simulink model "Control_Test"  (R2020a)
settings: Solver=ode1  StartTime=0.0  StopTime=inf  FixedStep=0.001  RelTol=1e-3
InitFcn:
  | COM_config;
  | IO_config;
values from neighbouring files (symbols this model uses):
  AirDensity_kgpm3 = 1.225    [vehicle_controller.mat]
  BatteryCapacity_Wh = 83    [vehicle_controller.mat]
  BatteryInitialEnergy = 58.1    [vehicle_controller.mat]
  BatteryMaxVoltage_V = 96    [vehicle_controller.mat]
  BatteryVoltageCoefficient_x = [0 0.1 0.2 0.3 0.4 0.5 0.6 0.7 0.8 0.9 1]    [vehicle_controller.mat]
  BatteryVoltageCoefficient_y = [0.833333333333 0.85 0.866666666667 0.883333333333 0.9 0.916666666667 0.933333333333 0.95 0.966666666667 0.983333333333 1]    [vehicle_controller.mat]
  BodyInitialSpeed_mps = 0    [vehicle_controller.mat]
  BodyMass_kg = 900    [vehicle_controller.mat]
  CombustionEngineMaxTorque_Nm = 100    [vehicle_controller.mat]
  DragArea_m2 = 4.5    [vehicle_controller.mat]
  DragCoeficient_1 = 0.4    [vehicle_controller.mat]
  FrictionCoefficient_Nsprad = 0.01    [vehicle_controller.mat]
  GearboxRatio_0_1 = 3    [vehicle_controller.mat]
  Ke = 0.1178    [vehicle_controller.mat]
  Kt = 0.668    [vehicle_controller.mat]
  L = looptransfer.Lo    [H_infinity_control_design.m]    (also in LoopShaping.m = G*K; Vehicle_Car_Controller.m = P * C)
  R = 0.141176    [vehicle_controller.mat]
  WheelDiameter_m = 0.5    [vehicle_controller.mat]
undefined symbols (not defined in the file or in its folder): AI_01_range, AI_02_range, AI_03_range, AI_04_range, AI_05_range, AI_06_range, AO_01_max, AO_02_max, AO_03_max, AO_04_max, AO_05_max, AO_06_max, Battery_Voltage_Req, DI_01_mode, DI_01_pullUpDown, DI_02_mode, DI_02_pullUpDown, DI_03_mode, DI_03_pullUpDown, DI_04_mode, DI_04_pullUpDown, DI_05_mode, DI_05_pullUpDown, DI_06_mode, DI_06_pullUpDown, DI_vref_threshold, DO_01_mode, DO_01_outStage, DO_02_mode, DO_02_outStage, DO_03_mode, DO_03_outStage, DO_04_mode, DO_04_outStage, DO_05_mode, DO_05_outStage, DO_06_mode, DO_06_outStage, DO_vref_high, package_period, Serial_Port, Standard_Devices
libraries: simulink x8, sldrtlib x2, simulink_extras x1
(part 2 of 2)

== system Control_Test/Config/Set2/0x1012 ==
  note: 6 Message IDs sent from device to calculator
      | ID 0 means: nothing else to send
  RollingCounter : Inport
  Data Type Conversion{,1..6} (7 alike) : DataTypeConversion
  Data1 : Constant  Value=0x2011
  Data2 : Constant  Value=0x2021
  Data3 : Constant  Value=0x2041
  Data4 : Constant  Value=0x2012
  Data5 : Constant  Value=0x2019
  Data6 : Constant  Value=0x2019
  ID : Constant  Value=0x1012
  Mux : Mux  Inputs=8
  PacketOut : Outport
  wires:
  Mux/1 -> PacketOut/1
  ID/1 -> Data Type Conversion6/1
  Data1/1 -> Data Type Conversion/1
  Data2/1 -> Data Type Conversion1/1
  Data3/1 -> Data Type Conversion2/1
  Data4/1 -> Data Type Conversion3/1
  Data5/1 -> Data Type Conversion4/1
  Data6/1 -> Data Type Conversion5/1
  RollingCounter/1 -> Mux/8
  Data Type Conversion/1 -> Mux/2
  Data Type Conversion1/1 -> Mux/3
  Data Type Conversion2/1 -> Mux/4
  Data Type Conversion3/1 -> Mux/5
  Data Type Conversion4/1 -> Mux/6
  Data Type Conversion5/1 -> Mux/7
  Data Type Conversion6/1 -> Mux/1

== system Control_Test/Config/Set2/0x1013 ==
  note: 6 Message IDs sent from device to calculator
      | ID 0 means: nothing else to send
  RollingCounter : Inport
  Data Type Conversion{,1..6} (7 alike) : DataTypeConversion
  Data1 : Constant  Value=0x2019
  Data2 : Constant  Value=0x2019
  Data{3..6} (4 alike) : Constant  Value=0
  ID : Constant  Value=0x1013
  Mux : Mux  Inputs=8
  PacketOut : Outport
  wires:
  RollingCounter/1 -> Mux/8
  Data6/1 -> Data Type Conversion5/1
  Data5/1 -> Data Type Conversion4/1
  Data4/1 -> Data Type Conversion3/1
  Data3/1 -> Data Type Conversion2/1
  Data2/1 -> Data Type Conversion1/1
  Data1/1 -> Data Type Conversion/1
  ID/1 -> Data Type Conversion6/1
  Mux/1 -> PacketOut/1
  Data Type Conversion5/1 -> Mux/7
  Data Type Conversion4/1 -> Mux/6
  Data Type Conversion3/1 -> Mux/5
  Data Type Conversion2/1 -> Mux/4
  Data Type Conversion1/1 -> Mux/3
  Data Type Conversion/1 -> Mux/2
  Data Type Conversion6/1 -> Mux/1

== system Control_Test/Config/Set2/0x1029 ==
  RollingCounter : Inport
  Data Type Conversion{,1..6} (7 alike) : DataTypeConversion
  Data1 : Constant  Value=AI_01_range
  Data2 : Constant  Value=AI_02_range
  Data3 : Constant  Value=AI_03_range
  Data4 : Constant  Value=AI_04_range
  Data5 : Constant  Value=AI_05_range
  Data6 : Constant  Value=AI_06_range
  ID : Constant  Value=0x1029
  Mux : Mux  Inputs=8
  PacketOut : Outport
  wires:
  Mux/1 -> PacketOut/1
  ID/1 -> Data Type Conversion6/1
  Data1/1 -> Data Type Conversion/1
  Data2/1 -> Data Type Conversion1/1
  Data3/1 -> Data Type Conversion2/1
  Data4/1 -> Data Type Conversion3/1
  Data5/1 -> Data Type Conversion4/1
  Data6/1 -> Data Type Conversion5/1
  RollingCounter/1 -> Mux/8
  Data Type Conversion5/1 -> Mux/7
  Data Type Conversion4/1 -> Mux/6
  Data Type Conversion3/1 -> Mux/5
  Data Type Conversion2/1 -> Mux/4
  Data Type Conversion1/1 -> Mux/3
  Data Type Conversion/1 -> Mux/2
  Data Type Conversion6/1 -> Mux/1

== system Control_Test/Config/Set2/0x1039 ==
  RollingCounter : Inport
  Data Type Conversion{,1..6} (7 alike) : DataTypeConversion
  Data1 : Constant  Value=AO_01_max
  Data2 : Constant  Value=AO_02_max
  Data3 : Constant  Value=AO_03_max
  Data4 : Constant  Value=AO_04_max
  Data5 : Constant  Value=AO_05_max
  Data6 : Constant  Value=AO_06_max
  ID : Constant  Value=0x1039
  Mux : Mux  Inputs=8
  PacketOut : Outport
  wires:
  RollingCounter/1 -> Mux/8
  Data6/1 -> Data Type Conversion5/1
  Data5/1 -> Data Type Conversion4/1
  Data4/1 -> Data Type Conversion3/1
  Data3/1 -> Data Type Conversion2/1
  Data2/1 -> Data Type Conversion1/1
  Data1/1 -> Data Type Conversion/1
  ID/1 -> Data Type Conversion6/1
  Mux/1 -> PacketOut/1
  Data Type Conversion5/1 -> Mux/7
  Data Type Conversion4/1 -> Mux/6
  Data Type Conversion3/1 -> Mux/5
  Data Type Conversion2/1 -> Mux/4
  Data Type Conversion1/1 -> Mux/3
  Data Type Conversion/1 -> Mux/2
  Data Type Conversion6/1 -> Mux/1

== system Control_Test/Config/Set2/0x1047 ==
  RollingCounter : Inport
  Data Type Conversion{,1..6} (7 alike) : DataTypeConversion
  Data1 : Constant  Value=DI_vref_threshold
  Data{2..6} (5 alike) : Constant  Value=0
  ID : Constant  Value=0x1047
  Mux : Mux  Inputs=8
  PacketOut : Outport
  wires:
  Mux/1 -> PacketOut/1
  ID/1 -> Data Type Conversion6/1
  Data1/1 -> Data Type Conversion/1
  Data2/1 -> Data Type Conversion1/1
  Data3/1 -> Data Type Conversion2/1
  Data4/1 -> Data Type Conversion3/1
  Data5/1 -> Data Type Conversion4/1
  Data6/1 -> Data Type Conversion5/1
  RollingCounter/1 -> Mux/8
  Data Type Conversion5/1 -> Mux/7
  Data Type Conversion4/1 -> Mux/6
  Data Type Conversion3/1 -> Mux/5
  Data Type Conversion2/1 -> Mux/4
  Data Type Conversion1/1 -> Mux/3
  Data Type Conversion/1 -> Mux/2
  Data Type Conversion6/1 -> Mux/1

== system Control_Test/Config/Set2/0x1048 ==
  RollingCounter : Inport
  Data Type Conversion{,1..6} (7 alike) : DataTypeConversion
  Data1 : Constant  Value=DI_01_pullUpDown
  Data2 : Constant  Value=DI_02_pullUpDown
  Data3 : Constant  Value=DI_03_pullUpDown
  Data4 : Constant  Value=DI_04_pullUpDown
  Data5 : Constant  Value=DI_05_pullUpDown
  Data6 : Constant  Value=DI_06_pullUpDown
  ID : Constant  Value=0x1048
  Mux : Mux  Inputs=8
  PacketOut : Outport
  wires:
  RollingCounter/1 -> Mux/8
  Data6/1 -> Data Type Conversion5/1
  Data5/1 -> Data Type Conversion4/1
  Data4/1 -> Data Type Conversion3/1
  Data3/1 -> Data Type Conversion2/1
  Data2/1 -> Data Type Conversion1/1
  Data1/1 -> Data Type Conversion/1
  ID/1 -> Data Type Conversion6/1
  Mux/1 -> PacketOut/1
  Data Type Conversion5/1 -> Mux/7
  Data Type Conversion4/1 -> Mux/6
  Data Type Conversion/1 -> Mux/2
  Data Type Conversion1/1 -> Mux/3
  Data Type Conversion2/1 -> Mux/4
  Data Type Conversion3/1 -> Mux/5
  Data Type Conversion6/1 -> Mux/1

== system Control_Test/Config/Set2/0x1049 ==
  RollingCounter : Inport
  Data Type Conversion{,1..6} (7 alike) : DataTypeConversion
  Data1 : Constant  Value=DI_01_mode
  Data2 : Constant  Value=DI_02_mode
  Data3 : Constant  Value=DI_03_mode
  Data4 : Constant  Value=DI_04_mode
  Data5 : Constant  Value=DI_05_mode
  Data6 : Constant  Value=DI_06_mode
  ID : Constant  Value=0x1049
  Mux : Mux  Inputs=8
  PacketOut : Outport
  wires:
  Mux/1 -> PacketOut/1
  ID/1 -> Data Type Conversion6/1
  Data1/1 -> Data Type Conversion/1
  Data2/1 -> Data Type Conversion1/1
  Data3/1 -> Data Type Conversion2/1
  Data4/1 -> Data Type Conversion3/1
  Data5/1 -> Data Type Conversion4/1
  Data6/1 -> Data Type Conversion5/1
  RollingCounter/1 -> Mux/8
  Data Type Conversion/1 -> Mux/2
  Data Type Conversion1/1 -> Mux/3
  Data Type Conversion2/1 -> Mux/4
  Data Type Conversion3/1 -> Mux/5
  Data Type Conversion4/1 -> Mux/6
  Data Type Conversion5/1 -> Mux/7
  Data Type Conversion6/1 -> Mux/1

== system Control_Test/Config/Set2/0x1058 ==
  RollingCounter : Inport
  Data Type Conversion{,1..6} (7 alike) : DataTypeConversion
  Data1 : Constant  Value=DO_vref_high
  Data{2..6} (5 alike) : Constant  Value=0
  ID : Constant  Value=0x1058
  Mux : Mux  Inputs=8
  PacketOut : Outport
  wires:
  RollingCounter/1 -> Mux/8
  Data6/1 -> Data Type Conversion5/1
  Data5/1 -> Data Type Conversion4/1
  Data4/1 -> Data Type Conversion3/1
  Data3/1 -> Data Type Conversion2/1
  Data2/1 -> Data Type Conversion1/1
  Data1/1 -> Data Type Conversion/1
  ID/1 -> Data Type Conversion6/1
  Mux/1 -> PacketOut/1
  Data Type Conversion/1 -> Mux/2
  Data Type Conversion1/1 -> Mux/3
  Data Type Conversion2/1 -> Mux/4
  Data Type Conversion3/1 -> Mux/5
  Data Type Conversion4/1 -> Mux/6
  Data Type Conversion5/1 -> Mux/7
  Data Type Conversion6/1 -> Mux/1

== system Control_Test/Config/Set3/0x1057 ==
  RollingCounter : Inport
  Data Type Conversion{1..7} (7 alike) : DataTypeConversion
  Data1 : Constant  Value=DO_01_outStage
  Data2 : Constant  Value=DO_02_outStage
  Data3 : Constant  Value=DO_03_outStage
  Data4 : Constant  Value=DO_04_outStage
  Data5 : Constant  Value=DO_05_outStage
  Data6 : Constant  Value=DO_06_outStage
  ID : Constant  Value=0x1057
  Mux : Mux  Inputs=8
  PacketOut : Outport
  wires:
  RollingCounter/1 -> Mux/8
  Data6/1 -> Data Type Conversion6/1
  Data5/1 -> Data Type Conversion5/1
  Data4/1 -> Data Type Conversion4/1
  Data3/1 -> Data Type Conversion3/1
  Data2/1 -> Data Type Conversion2/1
  Data1/1 -> Data Type Conversion1/1
  ID/1 -> Data Type Conversion7/1
  Mux/1 -> PacketOut/1
  Data Type Conversion4/1 -> Mux/5
  Data Type Conversion6/1 -> Mux/7
  Data Type Conversion2/1 -> Mux/3
  Data Type Conversion1/1 -> Mux/2
  Data Type Conversion3/1 -> Mux/4
  Data Type Conversion5/1 -> Mux/6
  Data Type Conversion7/1 -> Mux/1

== system Control_Test/Config/Set3/0x1059 ==
  RollingCounter : Inport
  Data Type Conversion{,1..6} (7 alike) : DataTypeConversion
  Data1 : Constant  Value=DO_01_mode
  Data2 : Constant  Value=DO_02_mode
  Data3 : Constant  Value=DO_03_mode
  Data4 : Constant  Value=DO_04_mode
  Data5 : Constant  Value=DO_05_mode
  Data6 : Constant  Value=DO_06_mode
  ID : Constant  Value=0x1059
  Mux : Mux  Inputs=8
  PacketOut : Outport
  wires:
  RollingCounter/1 -> Mux/8
  Data6/1 -> Data Type Conversion5/1
  Data5/1 -> Data Type Conversion4/1
  Data4/1 -> Data Type Conversion3/1
  Data3/1 -> Data Type Conversion2/1
  Data2/1 -> Data Type Conversion1/1
  Data1/1 -> Data Type Conversion/1
  ID/1 -> Data Type Conversion6/1
  Mux/1 -> PacketOut/1
  Data Type Conversion/1 -> Mux/2
  Data Type Conversion1/1 -> Mux/3
  Data Type Conversion2/1 -> Mux/4
  Data Type Conversion3/1 -> Mux/5
  Data Type Conversion4/1 -> Mux/6
  Data Type Conversion5/1 -> Mux/7
  Data Type Conversion6/1 -> Mux/1

== system Control_Test/Config/Set3/Empty2 ==
  RollingCounter : Inport
  Data Type Conversion{1..7} (7 alike) : DataTypeConversion
  Data{1..6} (6 alike) : Constant  Value=0
  ID : Constant  Value=0
  Mux : Mux  Inputs=8
  PacketOut : Outport
  wires:
  Data Type Conversion7/1 -> Mux/1
  Data Type Conversion5/1 -> Mux/6
  Data Type Conversion3/1 -> Mux/4
  Data Type Conversion1/1 -> Mux/2
  Data Type Conversion2/1 -> Mux/3
  Data Type Conversion6/1 -> Mux/7
  Data Type Conversion4/1 -> Mux/5
  Mux/1 -> PacketOut/1
  ID/1 -> Data Type Conversion7/1
  Data1/1 -> Data Type Conversion1/1
  Data2/1 -> Data Type Conversion2/1
  Data3/1 -> Data Type Conversion3/1
  Data4/1 -> Data Type Conversion4/1
  Data5/1 -> Data Type Conversion5/1
  Data6/1 -> Data Type Conversion6/1
  RollingCounter/1 -> Mux/8

== system Control_Test/Config/Set3/Empty3 ==
  RollingCounter : Inport
  Data Type Conversion{1..7} (7 alike) : DataTypeConversion
  Data{1..6} (6 alike) : Constant  Value=0
  ID : Constant  Value=0
  Mux : Mux  Inputs=8
  PacketOut : Outport
  wires:
  RollingCounter/1 -> Mux/8
  Data6/1 -> Data Type Conversion6/1
  Data5/1 -> Data Type Conversion5/1
  Data4/1 -> Data Type Conversion4/1
  Data3/1 -> Data Type Conversion3/1
  Data2/1 -> Data Type Conversion2/1
  Data1/1 -> Data Type Conversion1/1
  ID/1 -> Data Type Conversion7/1
  Mux/1 -> PacketOut/1
  Data Type Conversion4/1 -> Mux/5
  Data Type Conversion6/1 -> Mux/7
  Data Type Conversion2/1 -> Mux/3
  Data Type Conversion1/1 -> Mux/2
  Data Type Conversion3/1 -> Mux/4
  Data Type Conversion5/1 -> Mux/6
  Data Type Conversion7/1 -> Mux/1

== system Control_Test/Config/Set3/Empty4 ==
  RollingCounter : Inport
  Data Type Conversion{1..7} (7 alike) : DataTypeConversion
  Data{1..6} (6 alike) : Constant  Value=0
  ID : Constant  Value=0
  Mux : Mux  Inputs=8
  PacketOut : Outport
  wires:
  Data Type Conversion7/1 -> Mux/1
  Data Type Conversion5/1 -> Mux/6
  Data Type Conversion3/1 -> Mux/4
  Data Type Conversion1/1 -> Mux/2
  Data Type Conversion2/1 -> Mux/3
  Data Type Conversion6/1 -> Mux/7
  Data Type Conversion4/1 -> Mux/5
  Mux/1 -> PacketOut/1
  ID/1 -> Data Type Conversion7/1
  Data1/1 -> Data Type Conversion1/1
  Data2/1 -> Data Type Conversion2/1
  Data3/1 -> Data Type Conversion3/1
  Data4/1 -> Data Type Conversion4/1
  Data5/1 -> Data Type Conversion5/1
  Data6/1 -> Data Type Conversion6/1
  RollingCounter/1 -> Mux/8

== system Control_Test/Config/Set3/Empty5 ==
  RollingCounter : Inport
  Data Type Conversion{1..7} (7 alike) : DataTypeConversion
  Data{1..6} (6 alike) : Constant  Value=0
  ID : Constant  Value=0
  Mux : Mux  Inputs=8
  PacketOut : Outport
  wires:
  RollingCounter/1 -> Mux/8
  Data6/1 -> Data Type Conversion6/1
  Data5/1 -> Data Type Conversion5/1
  Data4/1 -> Data Type Conversion4/1
  Data3/1 -> Data Type Conversion3/1
  Data2/1 -> Data Type Conversion2/1
  Data1/1 -> Data Type Conversion1/1
  ID/1 -> Data Type Conversion7/1
  Mux/1 -> PacketOut/1
  Data Type Conversion4/1 -> Mux/5
  Data Type Conversion6/1 -> Mux/7
  Data Type Conversion2/1 -> Mux/3
  Data Type Conversion1/1 -> Mux/2
  Data Type Conversion3/1 -> Mux/4
  Data Type Conversion5/1 -> Mux/6
  Data Type Conversion7/1 -> Mux/1

== system Control_Test/Config/Set3/Empty6 ==
  RollingCounter : Inport
  Data Type Conversion{1..7} (7 alike) : DataTypeConversion
  Data{1..6} (6 alike) : Constant  Value=0
  ID : Constant  Value=0
  Mux : Mux  Inputs=8
  PacketOut : Outport
  wires:
  Data Type Conversion7/1 -> Mux/1
  Data Type Conversion5/1 -> Mux/6
  Data Type Conversion3/1 -> Mux/4
  Data Type Conversion1/1 -> Mux/2
  Data Type Conversion2/1 -> Mux/3
  Data Type Conversion6/1 -> Mux/7
  Data Type Conversion4/1 -> Mux/5
  Mux/1 -> PacketOut/1
  ID/1 -> Data Type Conversion7/1
  Data1/1 -> Data Type Conversion1/1
  Data2/1 -> Data Type Conversion2/1
  Data3/1 -> Data Type Conversion3/1
  Data4/1 -> Data Type Conversion4/1
  Data5/1 -> Data Type Conversion5/1
  Data6/1 -> Data Type Conversion6/1
  RollingCounter/1 -> Mux/8

== system Control_Test/Config/Set3/Empty7 ==
  RollingCounter : Inport
  Data Type Conversion{1..7} (7 alike) : DataTypeConversion
  Data{1..6} (6 alike) : Constant  Value=0
  ID : Constant  Value=0
  Mux : Mux  Inputs=8
  PacketOut : Outport
  wires:
  RollingCounter/1 -> Mux/8
  Data6/1 -> Data Type Conversion6/1
  Data5/1 -> Data Type Conversion5/1
  Data4/1 -> Data Type Conversion4/1
  Data3/1 -> Data Type Conversion3/1
  Data2/1 -> Data Type Conversion2/1
  Data1/1 -> Data Type Conversion1/1
  ID/1 -> Data Type Conversion7/1
  Mux/1 -> PacketOut/1
  Data Type Conversion4/1 -> Mux/5
  Data Type Conversion6/1 -> Mux/7
  Data Type Conversion2/1 -> Mux/3
  Data Type Conversion1/1 -> Mux/2
  Data Type Conversion3/1 -> Mux/4
  Data Type Conversion5/1 -> Mux/6
  Data Type Conversion7/1 -> Mux/1

== system Control_Test/Running/InSet/AI ==
  PacketIn : Inport
  Bus Creator : BusCreator  Inputs=6
  Demux : Demux  Outputs=8
  RollingCounter : Outport
  ID : Outport  Port=2
  AI : Outport  Port=3
  wires:
  Demux/7 -> Bus Creator/6  "AI_06"
  Demux/6 -> Bus Creator/5  "AI_05"
  Demux/5 -> Bus Creator/4  "AI_04"
  Demux/4 -> Bus Creator/3  "AI_03"
  Demux/3 -> Bus Creator/2  "AI_02"
  Demux/2 -> Bus Creator/1  "AI_01"
  Demux/1 -> ID/1
  Demux/8 -> RollingCounter/1
  PacketIn/1 -> Demux/1
  Bus Creator/1 -> AI/1

== system Control_Test/Running/InSet/BatteryVoltage ==
  PacketIn : Inport
  Demux : Demux  Outputs=8
  Terminator{1..5} (5 alike) : Terminator
  RollingCounter : Outport
  ID : Outport  Port=2
  Battery_Voltage : Outport  Port=3
  wires:
  Demux/7 -> Terminator5/1
  Demux/6 -> Terminator4/1
  Demux/5 -> Terminator3/1
  Demux/4 -> Terminator2/1
  Demux/3 -> Terminator1/1
  Demux/2 -> Battery_Voltage/1
  Demux/1 -> ID/1
  Demux/8 -> RollingCounter/1
  PacketIn/1 -> Demux/1

== system Control_Test/Running/InSet/DI ==
  PacketIn : Inport
  Bus Creator : BusCreator  Inputs=6
  Demux : Demux  Outputs=8
  RollingCounter : Outport
  ID : Outport  Port=2
  DI : Outport  Port=3
  wires:
  Bus Creator/1 -> DI/1
  PacketIn/1 -> Demux/1
  Demux/8 -> RollingCounter/1
  Demux/1 -> ID/1
  Demux/2 -> Bus Creator/1  "DI_01"
  Demux/3 -> Bus Creator/2  "DI_02"
  Demux/4 -> Bus Creator/3  "DI_03"
  Demux/5 -> Bus Creator/4  "DI_04"
  Demux/6 -> Bus Creator/5  "DI_05"
  Demux/7 -> Bus Creator/6  "DI_06"

== system Control_Test/Running/InSet/Empty2 ==
  PacketIn : Inport
  Demux : Demux  Outputs=8
  Terminator{,1..5} (6 alike) : Terminator
  RollingCounter : Outport
  ID : Outport  Port=2
  wires:
  Demux/7 -> Terminator5/1
  Demux/6 -> Terminator4/1
  Demux/5 -> Terminator3/1
  Demux/4 -> Terminator2/1
  Demux/3 -> Terminator1/1
  Demux/2 -> Terminator/1
  Demux/1 -> ID/1
  Demux/8 -> RollingCounter/1
  PacketIn/1 -> Demux/1

== system Control_Test/Running/InSet/Empty3 ==
  PacketIn : Inport
  Demux : Demux  Outputs=8
  Terminator{,1..5} (6 alike) : Terminator
  RollingCounter : Outport
  ID : Outport  Port=2
  wires:
  PacketIn/1 -> Demux/1
  Demux/8 -> RollingCounter/1
  Demux/1 -> ID/1
  Demux/2 -> Terminator/1
  Demux/3 -> Terminator1/1
  Demux/4 -> Terminator2/1
  Demux/5 -> Terminator3/1
  Demux/6 -> Terminator4/1
  Demux/7 -> Terminator5/1

== system Control_Test/Running/InSet/Empty4 ==
  PacketIn : Inport
  Demux : Demux  Outputs=8
  Terminator{,1..5} (6 alike) : Terminator
  RollingCounter : Outport
  ID : Outport  Port=2
  wires:
  PacketIn/1 -> Demux/1
  Demux/8 -> RollingCounter/1
  Demux/1 -> ID/1
  Demux/2 -> Terminator/1
  Demux/3 -> Terminator1/1
  Demux/4 -> Terminator2/1
  Demux/5 -> Terminator3/1
  Demux/6 -> Terminator4/1
  Demux/7 -> Terminator5/1

== system Control_Test/Running/InSet/Empty5 ==
  PacketIn : Inport
  Demux : Demux  Outputs=8
  Terminator{,1..5} (6 alike) : Terminator
  RollingCounter : Outport
  ID : Outport  Port=2
  wires:
  Demux/7 -> Terminator5/1
  Demux/6 -> Terminator4/1
  Demux/5 -> Terminator3/1
  Demux/4 -> Terminator2/1
  Demux/3 -> Terminator1/1
  Demux/2 -> Terminator/1
  Demux/1 -> ID/1
  Demux/8 -> RollingCounter/1
  PacketIn/1 -> Demux/1

== system Control_Test/Running/InSet/Empty6 ==
  PacketIn : Inport
  Demux : Demux  Outputs=8
  Terminator{,1..5} (6 alike) : Terminator
  RollingCounter : Outport
  ID : Outport  Port=2
  wires:
  Demux/7 -> Terminator5/1
  Demux/6 -> Terminator4/1
  Demux/5 -> Terminator3/1
  Demux/4 -> Terminator2/1
  Demux/3 -> Terminator1/1
  Demux/2 -> Terminator/1
  Demux/1 -> ID/1
  Demux/8 -> RollingCounter/1
  PacketIn/1 -> Demux/1

== system Control_Test/Running/Model/AirDrag ==
  VehicleSpeed_mps : Inport
  " " : Constant  Value=0.5
  AirDensity_kgpm3 : Constant  Value=AirDensity_kgpm3
  DragArea_m2 : Constant  Value=DragArea_m2
  DragCoeficient_1 : Constant  Value=DragCoeficient_1
  Product : Product  Inputs=5
  Square : Math  Operator=square  SaturateOnIntegerOverflow=on
  AirDragForce_N : Outport
  wires:
  VehicleSpeed_mps/1 -> Square/1
  Square/1 -> Product/5
  DragArea_m2/1 -> Product/3
  AirDensity_kgpm3/1 -> Product/4
  DragCoeficient_1/1 -> Product/2
  " "/1 -> Product/1
  Product/1 -> AirDragForce_N/1

== system Control_Test/Running/Model/Battery ==
  BatteryCurrent_A : Inport
  1-D Lookup Table : Lookup_n-D  NumberOfTableDimensions=1  BreakpointsForDimension1=BatteryVoltageCoefficient_x  Table=BatteryVoltageCoefficient_y  InternalRulePriority=Speed  RndMeth=Simplest  InputSameDT=on
  BatteryCapacity_Wh : Constant  Value=BatteryCapacity_Wh
  BatteryMaxVoltage_V : Constant  Value=BatteryMaxVoltage_V
  Gain : Gain  Gain=-1
  Gain1 : Gain  Gain=1/3600
  Integrator : Integrator  InitialCondition=BatteryInitialEnergy
  Product : Product
  Product1 : Product  Inputs=*/
  Product2 : Product
  BatteryVoltage_V : Outport
  wires:
  BatteryCurrent_A/1 -> Product2/1  "BatteryCurrent_A"
  Product/1 -> Product2/2, BatteryVoltage_V/1  "BatteryVoltage_V"
  Integrator/1 -> Product1/1  "Energy_Wh"
  1-D Lookup Table/1 -> Product/2  "VoltageCoeficient_0_1"
  BatteryMaxVoltage_V/1 -> Product/1
  BatteryCapacity_Wh/1 -> Product1/2
  Product1/1 -> 1-D Lookup Table/1  "StateOfCharge_0_1"
  Product2/1 -> Gain/1
  Gain/1 -> Gain1/1
  Gain1/1 -> Integrator/1

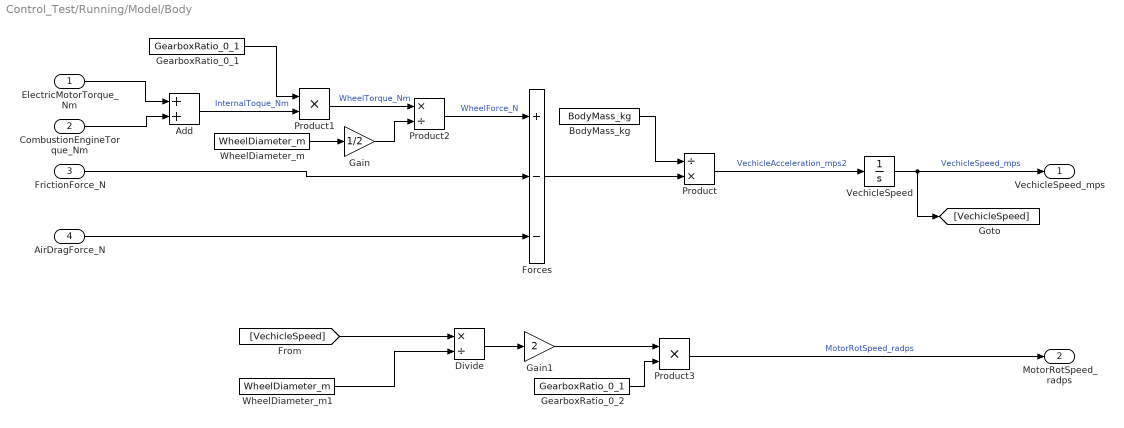
== system Control_Test/Running/Model/Body ==
  ElectricMotorTorque_Nm : Inport
  CombustionEngineTorque_Nm : Inport  Port=2
  FrictionForce_N : Inport  Port=3
  AirDragForce_N : Inport  Port=4
  Add : Sum
  BodyMass_kg : Constant  Value=BodyMass_kg
  Divide : Product  Inputs=*/
  Forces : Sum  Inputs=+--
  Gain : Gain  Gain=1/2
  Gain1 : Gain  Gain=2
  GearboxRatio_0_1 : Constant  Value=GearboxRatio_0_1
  GearboxRatio_0_2 : Constant  Value=GearboxRatio_0_1
  Product : Product  Inputs=/*
  Product1 : Product
  Product2 : Product  Inputs=*/
  Product3 : Product  Inputs=**
  VechicleSpeed : Integrator  InitialCondition=BodyInitialSpeed_mps
  WheelDiameter_m : Constant  Value=WheelDiameter_m
  WheelDiameter_m1 : Constant  Value=WheelDiameter_m
  VechicleSpeed_mps : Outport
  MotorRotSpeed_radps : Outport  Port=2
  wires:
  VechicleSpeed/1 -> [VechicleSpeed], VechicleSpeed_mps/1  "VechicleSpeed_mps"
  Product/1 -> VechicleSpeed/1  "VechicleAcceleration_mps2"
  BodyMass_kg/1 -> Product/1
  Forces/1 -> Product/2
  AirDragForce_N/1 -> Forces/3
  FrictionForce_N/1 -> Forces/2
  ElectricMotorTorque_Nm/1 -> Add/1
  CombustionEngineTorque_Nm/1 -> Add/2
  Add/1 -> Product1/2  "InternalToque_Nm"
  GearboxRatio_0_1/1 -> Product1/1
  Product1/1 -> Product2/1  "WheelTorque_Nm"
  WheelDiameter_m/1 -> Gain/1
  Product2/1 -> Forces/1  "WheelForce_N"
  Gain/1 -> Product2/2
  [VechicleSpeed] -> Divide/1
  WheelDiameter_m1/1 -> Divide/2
  Divide/1 -> Gain1/1
  Gain1/1 -> Product3/1
  GearboxRatio_0_2/1 -> Product3/2
  Product3/1 -> MotorRotSpeed_radps/1  "MotorRotSpeed_radps"

== system Control_Test/Running/Model/CombustionEngine ==
  CombustionEngineStart_1 : Inport
  Gain : Gain  Gain=CombustionEngineMaxTorque_Nm
  Transfer Fcn : TransferFcn  Denominator=[1 1]
  CombustionEngineTorque_Nm : Outport
  wires:
  Transfer Fcn/1 -> CombustionEngineTorque_Nm/1
  CombustionEngineStart_1/1 -> Gain/1
  Gain/1 -> Transfer Fcn/1

== system Control_Test/Running/Model/Driver ==
  BatteryVoltage_V : Inport
  DutyCycle_1 : Inport  Port=2
  Direction_1 : Inport  Port=3
  MotorCurrent_A : Inport  Port=4
  Product : Product
  Product1 : Product
  Product2 : Product
  MotorVoltage_V : Outport
  BatteryCurrent_A : Outport  Port=2
  wires:
  BatteryVoltage_V/1 -> Product/1
  Product/1 -> MotorVoltage_V/1
  Product2/1 -> Product1/1, Product/2
  MotorCurrent_A/1 -> Product1/2
  Product1/1 -> BatteryCurrent_A/1
  DutyCycle_1/1 -> Product2/1
  Direction_1/1 -> Product2/2

== system Control_Test/Running/Model/ElectricMotor ==
  MotorRotSpeed_radps : Inport
  MotorVoltage_V : Inport  Port=2
  Add : Sum  Inputs=-+-
  Constant : Constant  Value=Kt
  Constant1 : Constant  Value=L
  Constant2 : Constant  Value=R
  Constant3 : Constant  Value=Ke
  Integrator : Integrator
  Product : Product
  Product1 : Product  Inputs=*/
  Product2 : Product
  Product3 : Product
  Scope : Scope
  MotorTorque_Nm : Outport
  MotorCurrent_A : Outport  Port=2
  wires:
  Product/1 -> MotorTorque_Nm/1
  Integrator/1 -> MotorCurrent_A/1, Product2/2, Scope/1, Product/2  "MotorCurrent_A"
  Constant/1 -> Product/1
  Product1/1 -> Integrator/1
  Constant1/1 -> Product1/2
  Add/1 -> Product1/1
  Product2/1 -> Add/3
  Constant2/1 -> Product2/1
  MotorVoltage_V/1 -> Add/2
  Constant3/1 -> Product3/1
  Product3/1 -> Add/1
  MotorRotSpeed_radps/1 -> Product3/2

== system Control_Test/Running/Model/Frictions ==
  MotorSpeed_radps : Inport
  FrictionCoefficient_Nsprad : Constant  Value=FrictionCoefficient_Nsprad
  Product : Product
  FrictionForce_N : Outport
  wires:
  Product/1 -> FrictionForce_N/1
  MotorSpeed_radps/1 -> Product/2
  FrictionCoefficient_Nsprad/1 -> Product/1

== system Control_Test/Running/Model/Subsystem ==
  In1 : Inport
  Constant : Constant  Value=00  OutDataTypeStr=Inherit: Inherit via back propagation
  IsNaN : RelationalOperator  Operator=isNaN  OutDataTypeStr=boolean  RndMeth=Simplest
  Switch : Switch  Criteria=u2 > Threshold
  DutyCycle_1 : Outport
  wires:
  Switch/1 -> DutyCycle_1/1
  In1/1 -> IsNaN/1, Switch/3
  IsNaN/1 -> Switch/2
  Constant/1 -> Switch/1

== system Control_Test/Running/Model/Subsystem1 ==
  In1 : Inport
  Constant : Constant  Value=00  OutDataTypeStr=Inherit: Inherit via back propagation
  IsNaN : RelationalOperator  Operator=isNaN  OutDataTypeStr=boolean  RndMeth=Simplest
  Switch : Switch  Criteria=u2 > Threshold
  Direction_1 : Outport
  wires:
  Constant/1 -> Switch/1
  IsNaN/1 -> Switch/2
  In1/1 -> Switch/3, IsNaN/1
  Switch/1 -> Direction_1/1

== system Control_Test/Running/Model/Subsystem2 ==
  In1 : Inport
  Constant : Constant  Value=00  OutDataTypeStr=Inherit: Inherit via back propagation
  IsNaN : RelationalOperator  Operator=isNaN  OutDataTypeStr=boolean  RndMeth=Simplest
  Switch : Switch  Criteria=u2 > Threshold
  Direction_1 : Outport
  wires:
  Switch/1 -> Direction_1/1
  In1/1 -> IsNaN/1, Switch/3
  IsNaN/1 -> Switch/2
  Constant/1 -> Switch/1

== system Control_Test/Running/ModelInputs/Subsystem2 ==
  <AI> : Inport
  Bus Selector1 : BusSelector  OutputSignals=AI_01,AI_02,AI_03,AI_04,AI_05,AI_06
  Data Type Conversion{,1..5} (6 alike) : DataTypeConversion
  tag scope: AI_01=scoped, AI_02=scoped, AI_03=scoped, AI_04=scoped, AI_05=scoped, AI_06=scoped
  wires:
  Bus Selector1/4 -> Data Type Conversion3/1  "<AI_04>"
  Bus Selector1/3 -> Data Type Conversion2/1  "<AI_03>"
  Bus Selector1/6 -> Data Type Conversion5/1  "<AI_06>"
  Bus Selector1/2 -> Data Type Conversion1/1  "<AI_02>"
  Bus Selector1/1 -> Data Type Conversion/1  "<AI_01>"
  <AI>/1 -> Bus Selector1/1
  Data Type Conversion/1 -> [AI_01]
  Bus Selector1/5 -> Data Type Conversion4/1  "<AI_05>"
  Data Type Conversion1/1 -> [AI_02]
  Data Type Conversion2/1 -> [AI_03]
  Data Type Conversion3/1 -> [AI_04]
  Data Type Conversion4/1 -> [AI_05]
  Data Type Conversion5/1 -> [AI_06]

== system Control_Test/Running/ModelInputs/Subsystem3 ==
  <DI> : Inport
  Bus Selector2 : BusSelector  OutputSignals=DI_01,DI_02,DI_03,DI_04,DI_05,DI_06
  Data Type Conversion{,1..5} (6 alike) : DataTypeConversion
  tag scope: DI_01=scoped, DI_02=scoped, DI_03=scoped, DI_04=scoped, DI_05=scoped, DI_06=scoped
  wires:
  Bus Selector2/3 -> Data Type Conversion2/1  "<DI_03>"
  Bus Selector2/6 -> Data Type Conversion5/1  "<DI_06>"
  Bus Selector2/2 -> Data Type Conversion1/1  "<DI_02>"
  Bus Selector2/1 -> Data Type Conversion/1  "<DI_01>"
  Bus Selector2/4 -> Data Type Conversion3/1  "<DI_04>"
  Bus Selector2/5 -> Data Type Conversion4/1  "<DI_05>"
  <DI>/1 -> Bus Selector2/1
  Data Type Conversion/1 -> [DI_01]
  Data Type Conversion3/1 -> [DI_04]
  Data Type Conversion4/1 -> [DI_05]
  Data Type Conversion5/1 -> [DI_06]
  Data Type Conversion1/1 -> [DI_02]
  Data Type Conversion2/1 -> [DI_03]

== system Control_Test/Running/ModelOutputs/AO ==
  Bus Creator : BusCreator  Inputs=6
  Data Type Conversion{,1..5} (6 alike) : DataTypeConversion  OutDataTypeStr=uint32
  AO : Outport
  wires:
  Data Type Conversion1/1 -> Bus Creator/2  "AO_02"
  Data Type Conversion3/1 -> Bus Creator/4  "AO_04"
  Data Type Conversion4/1 -> Bus Creator/5  "AO_05"
  [AO_06] -> Data Type Conversion5/1  "AO_06"
  Data Type Conversion2/1 -> Bus Creator/3  "AO_03"
  Data Type Conversion/1 -> Bus Creator/1  "AO_01"
  Bus Creator/1 -> AO/1  "AO"
  Data Type Conversion5/1 -> Bus Creator/6  "AO_06"
  [AO_05] -> Data Type Conversion4/1  "AO_05"
  [AO_01] -> Data Type Conversion/1  "AO_01"
  [AO_02] -> Data Type Conversion1/1  "AO_02"
  [AO_03] -> Data Type Conversion2/1  "AO_03"
  [AO_04] -> Data Type Conversion3/1  "AO_04"

== system Control_Test/Running/ModelOutputs/DO_Duty ==
  Bus Creator3 : BusCreator  Inputs=6
  Data Type Conversion{,1..5} (6 alike) : DataTypeConversion  OutDataTypeStr=uint32
  DO_Duty : Outport
  wires:
  Data Type Conversion1/1 -> Bus Creator3/2  "DO_02_Duty"
  Data Type Conversion5/1 -> Bus Creator3/6  "DO_06_Duty"
  Data Type Conversion/1 -> Bus Creator3/1  "DO_01_Duty"
  Data Type Conversion4/1 -> Bus Creator3/5  "DO_05_Duty"
  Data Type Conversion2/1 -> Bus Creator3/3  "DO_03_Duty"
  Data Type Conversion3/1 -> Bus Creator3/4  "DO_04_Duty"
  Bus Creator3/1 -> DO_Duty/1  "DO_Duty"
  [DO_01_Duty] -> Data Type Conversion/1  "DO_01_Duty"
  [DO_02_Duty] -> Data Type Conversion1/1  "DO_02_Duty"
  [DO_03_Duty] -> Data Type Conversion2/1  "DO_03_Duty"
  [DO_04_Duty] -> Data Type Conversion3/1  "DO_04_Duty"
  [DO_05_Duty] -> Data Type Conversion4/1  "DO_05_Duty"
  [DO_06_Duty] -> Data Type Conversion5/1  "DO_06_Duty"

== system Control_Test/Running/ModelOutputs/DO_Freq ==
  Bus Creator2 : BusCreator  Inputs=6
  Data Type Conversion{,1..5} (6 alike) : DataTypeConversion  OutDataTypeStr=uint32
  DO_Freq : Outport
  wires:
  Data Type Conversion/1 -> Bus Creator2/1  "DO_01_Freq"
  Data Type Conversion3/1 -> Bus Creator2/4  "DO_04_Freq"
  Bus Creator2/1 -> DO_Freq/1  "DO_Freq"
  Data Type Conversion4/1 -> Bus Creator2/5  "DO_05_Freq"
  Data Type Conversion5/1 -> Bus Creator2/6  "DO_06_Freq"
  Data Type Conversion2/1 -> Bus Creator2/3  "DO_03_Freq"
  Data Type Conversion1/1 -> Bus Creator2/2  "DO_02_Freq"
  [DO_01_Freq] -> Data Type Conversion/1  "DO_01_Freq"
  [DO_02_Freq] -> Data Type Conversion1/1  "DO_02_Freq"
  [DO_03_Freq] -> Data Type Conversion2/1  "DO_03_Freq"
  [DO_04_Freq] -> Data Type Conversion3/1  "DO_04_Freq"
  [DO_05_Freq] -> Data Type Conversion4/1  "DO_05_Freq"
  [DO_06_Freq] -> Data Type Conversion5/1  "DO_06_Freq"

== system Control_Test/Running/ModelOutputs/DO_Level ==
  Bus Creator1 : BusCreator  Inputs=6
  Data Type Conversion{,1..5} (6 alike) : DataTypeConversion  OutDataTypeStr=uint32
  DO_Level : Outport
  wires:
  Data Type Conversion1/1 -> Bus Creator1/2  "DO_02_Level"
  Bus Creator1/1 -> DO_Level/1  "DO_Level"
  Data Type Conversion2/1 -> Bus Creator1/3  "DO_03_Level"
  Data Type Conversion4/1 -> Bus Creator1/5  "DO_05_Level"
  Data Type Conversion3/1 -> Bus Creator1/4  "DO_04_Level"
  Data Type Conversion/1 -> Bus Creator1/1  "DO_01_Level"
  Data Type Conversion5/1 -> Bus Creator1/6  "DO_06_Level"
  [DO_04] -> Data Type Conversion3/1  "DO_04_Level"
  [DO_03] -> Data Type Conversion2/1  "DO_03_Level"
  [DO_02] -> Data Type Conversion1/1  "DO_02_Level"
  [DO_01] -> Data Type Conversion/1  "DO_01_Level"
  [DO_05] -> Data Type Conversion4/1  "DO_05_Level"
  [DO_06] -> Data Type Conversion5/1  "DO_06_Level"

== system Control_Test/Running/OutSet/0x1019 ==
  RollingCounter : Inport
  Battery_Active : Inport  Port=2
  Data Type Conversion{1..7} (7 alike) : DataTypeConversion
  Data2 : Constant  Value=Battery_Voltage_Req
  Data{3..6} (4 alike) : Constant  Value=0
  ID : Constant  Value=0x1019
  Mux : Mux  Inputs=8
  PacketOut : Outport
  wires:
  RollingCounter/1 -> Mux/8
  Data6/1 -> Data Type Conversion6/1
  Data5/1 -> Data Type Conversion5/1
  Data4/1 -> Data Type Conversion4/1
  Data3/1 -> Data Type Conversion3/1
  Data2/1 -> Data Type Conversion2/1
  Battery_Active/1 -> Data Type Conversion1/1
  ID/1 -> Data Type Conversion7/1
  Mux/1 -> PacketOut/1
  Data Type Conversion4/1 -> Mux/5
  Data Type Conversion6/1 -> Mux/7
  Data Type Conversion2/1 -> Mux/3
  Data Type Conversion1/1 -> Mux/2
  Data Type Conversion3/1 -> Mux/4
  Data Type Conversion5/1 -> Mux/6
  Data Type Conversion7/1 -> Mux/1

== system Control_Test/Running/OutSet/0x1031 ==
  RollingCounter : Inport
  DAC : Inport  Port=2
  Bus Selector : BusSelector  OutputSignals=AO_01,AO_02,AO_03,AO_04,AO_05,AO_06
  ID : Constant  Value=0x1031  OutDataTypeStr=uint32
  Mux : Mux  Inputs=8
  PacketOut : Outport
  wires:
  Mux/1 -> PacketOut/1
  ID/1 -> Mux/1
  RollingCounter/1 -> Mux/8
  DAC/1 -> Bus Selector/1
  Bus Selector/1 -> Mux/2  "<AO_01>"
  Bus Selector/2 -> Mux/3  "<AO_02>"
  Bus Selector/3 -> Mux/4  "<AO_03>"
  Bus Selector/4 -> Mux/5  "<AO_04>"
  Bus Selector/5 -> Mux/6  "<AO_05>"
  Bus Selector/6 -> Mux/7  "<AO_06>"

== system Control_Test/Running/OutSet/0x1051 ==
  RollingCounter : Inport
  DO_Level : Inport  Port=2
  Bus Selector : BusSelector  OutputSignals=DO_01_Level,DO_02_Level,DO_03_Level,DO_04_Level,DO_05_Level,DO_06_Level
  ID : Constant  Value=0x1051  OutDataTypeStr=uint32
  Mux : Mux  Inputs=8
  PacketOut : Outport
  wires:
  RollingCounter/1 -> Mux/8
  Bus Selector/5 -> Mux/6  "<DO_05_Level>"
  Bus Selector/3 -> Mux/4  "<DO_03_Level>"
  Bus Selector/1 -> Mux/2  "<DO_01_Level>"
  ID/1 -> Mux/1
  Mux/1 -> PacketOut/1
  DO_Level/1 -> Bus Selector/1
  Bus Selector/2 -> Mux/3  "<DO_02_Level>"
  Bus Selector/4 -> Mux/5  "<DO_04_Level>"
  Bus Selector/6 -> Mux/7  "<DO_06_Level>"

== system Control_Test/Running/OutSet/0x1052 ==
  RollingCounter : Inport
  DO_Freq : Inport  Port=2
  Bus Selector : BusSelector  OutputSignals=DO_01_Freq,DO_02_Freq,DO_03_Freq,DO_04_Freq,DO_05_Freq,DO_06_Freq
  ID : Constant  Value=0x1052  OutDataTypeStr=uint32
  Mux : Mux  Inputs=8
  PacketOut : Outport
  wires:
  Mux/1 -> PacketOut/1
  ID/1 -> Mux/1
  RollingCounter/1 -> Mux/8
  DO_Freq/1 -> Bus Selector/1
  Bus Selector/1 -> Mux/2  "<DO_01_Freq>"
  Bus Selector/2 -> Mux/3  "<DO_02_Freq>"
  Bus Selector/3 -> Mux/4  "<DO_03_Freq>"
  Bus Selector/4 -> Mux/5  "<DO_04_Freq>"
  Bus Selector/5 -> Mux/6  "<DO_05_Freq>"
  Bus Selector/6 -> Mux/7  "<DO_06_Freq>"

== system Control_Test/Running/OutSet/0x1053 ==
  RollingCounter : Inport
  DO_Duty : Inport  Port=2
  Bus Selector : BusSelector  OutputSignals=DO_01_Duty,DO_02_Duty,DO_03_Duty,DO_04_Duty,DO_05_Duty,DO_06_Duty
  ID : Constant  Value=0x1053  OutDataTypeStr=uint32
  Mux : Mux  Inputs=8
  PacketOut : Outport
  wires:
  RollingCounter/1 -> Mux/8
  ID/1 -> Mux/1
  Mux/1 -> PacketOut/1
  DO_Duty/1 -> Bus Selector/1
  Bus Selector/1 -> Mux/2  "<DO_01_Duty>"
  Bus Selector/2 -> Mux/3  "<DO_02_Duty>"
  Bus Selector/3 -> Mux/4  "<DO_03_Duty>"
  Bus Selector/4 -> Mux/5  "<DO_04_Duty>"
  Bus Selector/5 -> Mux/6  "<DO_05_Duty>"
  Bus Selector/6 -> Mux/7  "<DO_06_Duty>"

== system Control_Test/Running/OutSet/Empty2 ==
  RollingCounter : Inport
  Data Type Conversion{1..7} (7 alike) : DataTypeConversion
  Data{1..6} (6 alike) : Constant  Value=0
  ID : Constant  Value=0
  Mux : Mux  Inputs=8
  PacketOut : Outport
  wires:
  Data Type Conversion7/1 -> Mux/1
  Data Type Conversion5/1 -> Mux/6
  Data Type Conversion3/1 -> Mux/4
  Data Type Conversion1/1 -> Mux/2
  Data Type Conversion2/1 -> Mux/3
  Data Type Conversion6/1 -> Mux/7
  Data Type Conversion4/1 -> Mux/5
  Mux/1 -> PacketOut/1
  ID/1 -> Data Type Conversion7/1
  Data1/1 -> Data Type Conversion1/1
  Data2/1 -> Data Type Conversion2/1
  Data3/1 -> Data Type Conversion3/1
  Data4/1 -> Data Type Conversion4/1
  Data5/1 -> Data Type Conversion5/1
  Data6/1 -> Data Type Conversion6/1
  RollingCounter/1 -> Mux/8

== system Control_Test/Running/OutSet/Empty3 ==
  RollingCounter : Inport
  Data Type Conversion{1..7} (7 alike) : DataTypeConversion
  Data{1..6} (6 alike) : Constant  Value=0
  ID : Constant  Value=0
  Mux : Mux  Inputs=8
  PacketOut : Outport
  wires:
  RollingCounter/1 -> Mux/8
  Data6/1 -> Data Type Conversion6/1
  Data5/1 -> Data Type Conversion5/1
  Data4/1 -> Data Type Conversion4/1
  Data3/1 -> Data Type Conversion3/1
  Data2/1 -> Data Type Conversion2/1
  Data1/1 -> Data Type Conversion1/1
  ID/1 -> Data Type Conversion7/1
  Mux/1 -> PacketOut/1
  Data Type Conversion4/1 -> Mux/5
  Data Type Conversion6/1 -> Mux/7
  Data Type Conversion2/1 -> Mux/3
  Data Type Conversion1/1 -> Mux/2
  Data Type Conversion3/1 -> Mux/4
  Data Type Conversion5/1 -> Mux/6
  Data Type Conversion7/1 -> Mux/1

== system Control_Test/Running/OutSet/Empty4 ==
  RollingCounter : Inport
  Data Type Conversion{1..7} (7 alike) : DataTypeConversion
  Data{1..6} (6 alike) : Constant  Value=0
  ID : Constant  Value=0
  Mux : Mux  Inputs=8
  PacketOut : Outport
  wires:
  Data Type Conversion7/1 -> Mux/1
  Data Type Conversion5/1 -> Mux/6
  Data Type Conversion3/1 -> Mux/4
  Data Type Conversion1/1 -> Mux/2
  Data Type Conversion2/1 -> Mux/3
  Data Type Conversion6/1 -> Mux/7
  Data Type Conversion4/1 -> Mux/5
  Mux/1 -> PacketOut/1
  ID/1 -> Data Type Conversion7/1
  Data1/1 -> Data Type Conversion1/1
  Data2/1 -> Data Type Conversion2/1
  Data3/1 -> Data Type Conversion3/1
  Data4/1 -> Data Type Conversion4/1
  Data5/1 -> Data Type Conversion5/1
  Data6/1 -> Data Type Conversion6/1
  RollingCounter/1 -> Mux/8
